simulink model "FlightSimulation"  (R2023b)
settings: Solver=VariableStepAuto  StartTime=0.0  StopTime=10.0  RelTol=1e-3
values from neighbouring files (symbols this model uses):
  simCfg =     [matlab.mat]
settings Model: Creator=Blind  LastModifiedBy=frostydev
settings RTWCC: GPUComputeCapability=5.0

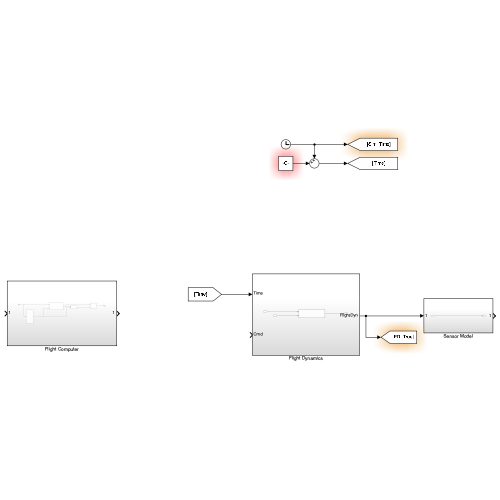
[thumbnail: Simulink's stored preview of the top-level diagram]
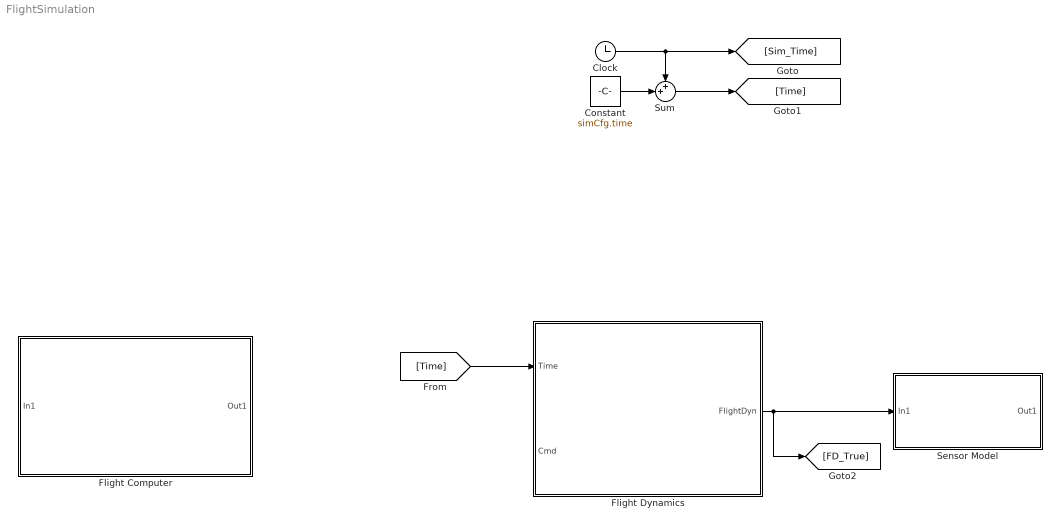
== system FlightSimulation ==
  Clock : Clock
  Constant : Constant  Value=simCfg.time
  Flight Computer : Subsystem
  Flight Dynamics : Subsystem
  Sensor Model : Subsystem
  Sum : Sum  Inputs=++|
  wires:
  Clock/1 -> Sum/1, [Sim_Time]
  Constant/1 -> Sum/2
  Sum/1 -> [Time]
  [Time] -> Flight Dynamics/1(Time)
  Flight Dynamics/1(FlightDyn) -> [FD_True], Sensor Model/1(In1)

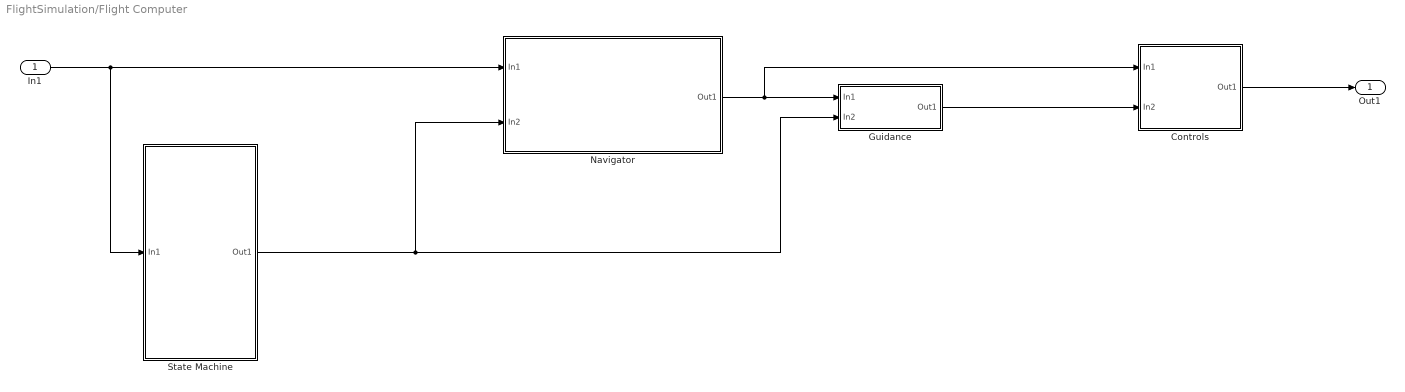
== system FlightSimulation/Flight Computer ==
  In1 : Inport
  Controls : Subsystem
  Guidance : Subsystem
  Navigator : Subsystem
  State Machine : Subsystem
  Out1 : Outport
  wires:
  In1/1 -> Navigator/1(In1), State Machine/1(In1)
  Guidance/1(Out1) -> Controls/2(In2)
  Navigator/1(Out1) -> Controls/1(In1), Guidance/1(In1)
  State Machine/1(Out1) -> Guidance/2(In2), Navigator/2(In2)
  Controls/1(Out1) -> Out1/1

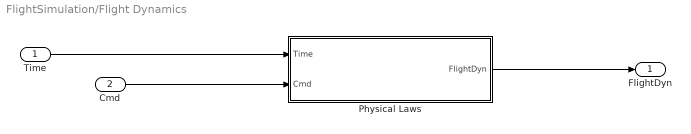
== system FlightSimulation/Flight Dynamics ==
  Time : Inport
  Cmd : Inport  Port=2
  Physical Laws : Subsystem
  FlightDyn : Outport
  wires:
  Cmd/1 -> Physical Laws/2(Cmd)
  Time/1 -> Physical Laws/1(Time)
  Physical Laws/1(FlightDyn) -> FlightDyn/1

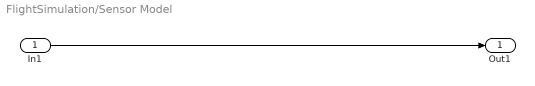
== system FlightSimulation/Sensor Model ==
  In1 : Inport
  Out1 : Outport
  wires:
  In1/1 -> Out1/1

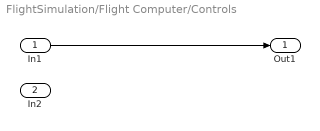
== system FlightSimulation/Flight Computer/Controls ==
  In1 : Inport
  In2 : Inport  Port=2
  Out1 : Outport
  wires:
  In1/1 -> Out1/1

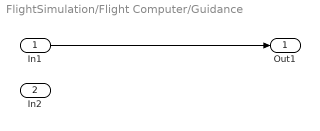
== system FlightSimulation/Flight Computer/Guidance ==
  In1 : Inport
  In2 : Inport  Port=2
  Out1 : Outport
  wires:
  In1/1 -> Out1/1

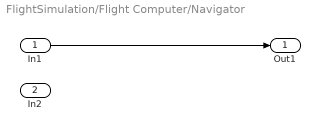
== system FlightSimulation/Flight Computer/Navigator ==
  In1 : Inport
  In2 : Inport  Port=2
  Out1 : Outport
  wires:
  In1/1 -> Out1/1

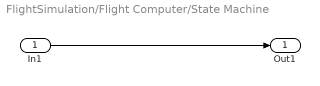
== system FlightSimulation/Flight Computer/State Machine ==
  In1 : Inport
  Out1 : Outport
  wires:
  In1/1 -> Out1/1

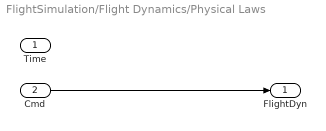
== system FlightSimulation/Flight Dynamics/Physical Laws ==
  Time : Inport
  Cmd : Inport  Port=2
  FlightDyn : Outport
  wires:
  Cmd/1 -> FlightDyn/1
